simulink model "uarttest"  (R2025a)
settings: Solver=VariableStepAuto  StartTime=0.0  StopTime=10.0  RelTol=1e-3
libraries: frdmk64flib x1
settings Model: Creator=ybakr  LastModifiedBy=ybakr

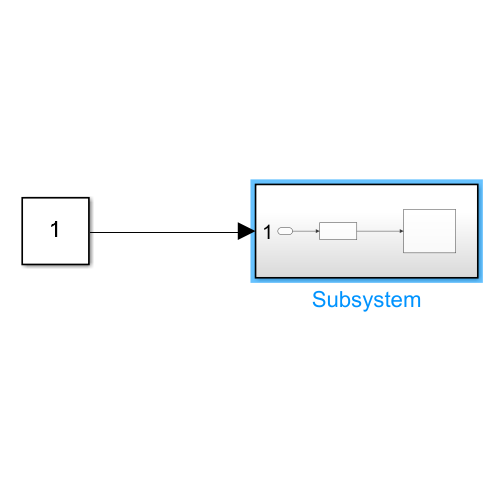
[thumbnail: Simulink's stored preview of the top-level diagram]
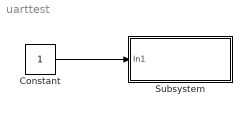
== system uarttest ==
  Constant : Constant
  Subsystem : Subsystem
  wires:
  Constant/1 -> Subsystem/1(In1)

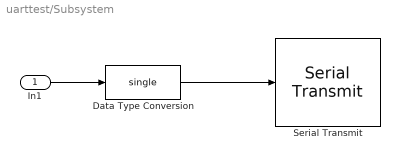
== system uarttest/Subsystem ==
  In1 : Inport
  Data Type Conversion : DataTypeConversion  OutDataTypeStr=single  SaturateOnIntegerOverflow=off  RndMeth=Floor
  Serial Transmit : frdmk64flib/Serial Transmit  SCIModule=0  Baudrate=uint32(9600)  Parity=None  StopBits=1  HardwareFlowControl=None  ByteOrder=LittleEndian  BlockingMode=on  OutputStatus=off
  wires:
  In1/1 -> Data Type Conversion/1
  Data Type Conversion/1 -> Serial Transmit/1
